simulink model "schema_robot_CT"  (R2017a)
settings: Solver=VariableStepAuto  StartTime=0.0  StopTime=10.0  RelTol=1e-3  EnableMultiTasking=on
values from neighbouring files (symbols this model uses):
  RB = struct()    [robot_numeric.m]    (also in robot_numeric_2.m)
settings Model: Creator=ygorra  LastModifiedBy=planusse
settings OptimizationCC: LifeSpan=inf
settings DebuggingCC: SFUnexpectedBacktrackingDiag=warning  SFNoUnconditionalDefaultTransitionDiag=warning  SFExecutionAtInitializationDiag=none
settings GRTTargetCC: TargetLangStandard=C89/C90 (ANSI)  GeneratePreprocessorConditionals=Disable all
settings ConfigComp: CovMetricSettings=dw  CovHtmlReporting=on  CovSaveCumulativeToWorkspaceVar=on  CovSaveSingleToWorkspaceVar=on  CovExternalEMLEnable=off

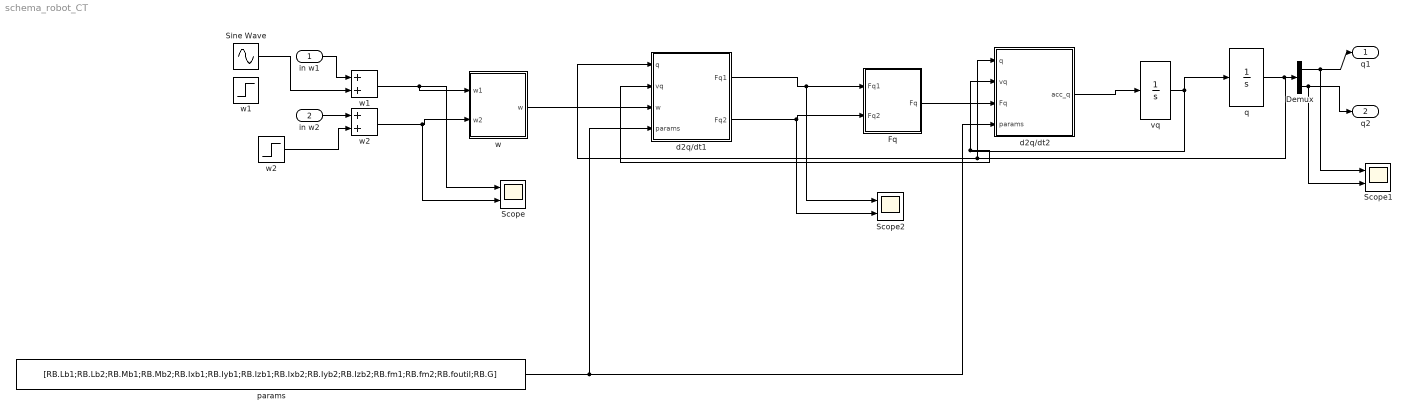
== system schema_robot_CT ==
  in w1 : Inport
  in w2 : Inport  Port=2
  Demux : Demux  Outputs=2
  Fq : MATLAB Function  TreatAsAtomicUnit=on
  Scope : Scope  NumInputPorts=2
  Scope1 : Scope  NumInputPorts=2
  Scope2 : Scope  NumInputPorts=2
  Sine Wave : Sin  Amplitude=0.1  SampleTime=0
  d2q/dt1 : MATLAB Function  TreatAsAtomicUnit=on
  d2q/dt2 : MATLAB Function  TreatAsAtomicUnit=on
  params : Constant  Value=[RB.Lb1;RB.Lb2;RB.Mb1;RB.Mb2;RB.Ixb1;RB.Iyb1;RB.Izb1;RB.Ixb2;RB.Iyb2;RB.Izb2;RB.fm1;RB.fm2;RB.foutil;RB.G]
  q : Integrator  InitialCondition=[RB.q1_init;RB.q2_init]  ContinuousStateAttributes='q'
  vq : Integrator  InitialCondition=[RB.vq1_init;RB.vq2_init]  ContinuousStateAttributes='vq'
  w : MATLAB Function  TreatAsAtomicUnit=on
  "w1  " : Step  Time=RB.t_Fq1  Before=RB.Fq1_0  After=RB.Fq1_1  SampleTime=0
  "w1   " : Sum
  "w2 " : Step  Time=RB.t_Fq2  Before=RB.Fq2_0  After=RB.Fq2_1  SampleTime=0
  "w2   " : Sum
  q1 : Outport
  q2 : Outport  Port=2
  wires:
  Demux/1 -> Scope1/1, q1/1
  d2q/dt2/1(acc_q) -> vq/1
  vq/1 -> d2q/dt1/2(vq), d2q/dt2/2(vq), q/1
  q/1 -> Demux/1, d2q/dt1/1(q), d2q/dt2/1(q)
  Fq/1(Fq) -> d2q/dt2/3(Fq)
  params/1 -> d2q/dt1/4(params), d2q/dt2/4(params)
  in w1/1 -> "w1   "/1
  in w2/1 -> "w2   "/1
  "w2 "/1 -> "w2   "/2
  Demux/2 -> Scope1/2, q2/1
  d2q/dt1/1(Fq1) -> Scope2/1, Fq/1(Fq1)
  d2q/dt1/2(Fq2) -> Scope2/2, Fq/2(Fq2)
  w/1(w) -> d2q/dt1/3(w)
  "w1   "/1 -> w/1(w1), Scope/1
  "w2   "/1 -> Scope/2, w/2(w2)
  Sine Wave/1 -> "w1   "/2

== matlab function schema_robot_CT/Fq ==
  data: Fq1 input; Fq2 input; Fq output
function Fq=Fq_(Fq1,Fq2)
    Fq=[Fq1;Fq2];
end

== matlab function schema_robot_CT/d2q//dt2 ==
  data: q input; vq input; Fq input; acc_q output; params input
function acc_q=clc_accq(q,vq,Fq,params)
    q1=q(1);    
    q2=q(2);
    vq1=vq(1);
    vq2=vq(2);
    Lb1=params(1);
    Lb2=params(2);
    Mb1=params(3);
    Mb2=params(4);
    Ixb1=params(5);
    Iyb1=params(6);
    Izb1=params(7);
    Ixb2=params(8);
    Iyb2=params(9);
    Izb2=params(10);
    fm1=params(11);
    fm2=params(12);
    foutil=params(13);
    G=params(14);
    A= clc_A(q1,q2,Lb1,Lb2,Mb1,Mb2,Ixb1,Iyb1,Izb1,Ixb2,Iyb2,Izb2,fm1,fm2,foutil,G);
    H= clc_H(q1,q2,vq1,vq2,Lb1,Lb2,Mb1,Mb2,Ixb1,Iyb1,Izb1,Ixb2,Iyb2,Izb2,fm1,fm2,foutil,G);
    acc_q=pinv(A)*(Fq-H);
end

== matlab function schema_robot_CT/d2q//dt1 ==
  data: q input; vq input; w input; Fq1 output; params input; Fq2 output
function [Fq1,Fq2]=clc_CT(q,vq,w,params)
q1=q(1);
q2=q(2);
vq1=vq(1);
vq2=vq(2);
Lb1=params(1);
Lb2=params(2);
Mb1=params(3);
Mb2=params(4);
Ixb1=params(5);
Iyb1=params(6);
Izb1=params(7);
Ixb2=params(8);
Iyb2=params(9);
Izb2=params(10);
fm1=params(11);
fm2=params(12);
foutil=params(13);
G=params(14);
A= clc_A(q1,q2,Lb1,Lb2,Mb1,Mb2,Ixb1,Iyb1,Izb1,Ixb2,Iyb2,Izb2,fm1,fm2,foutil,G);
H= clc_H(q1,q2,vq1,vq2,Lb1,Lb2,Mb1,Mb2,Ixb1,Iyb1,Izb1,Ixb2,Iyb2,Izb2,fm1,fm2,foutil,G);
Fq=A*w+H;
Fq1=Fq(1);
Fq2=Fq(2);
end

== matlab function schema_robot_CT/w ==
  data: w1 input; w2 input; w output
function w= w(w1,w2)
    w=[w1;w2];
end
